simulink model "variable_window_size_alg_1"  (R2019b)
settings: Solver=ode45  StartTime=0.0  StopTime=3  MaxStep=1e-4  RelTol=1e-4  AbsTol=1e-6
values from neighbouring files (symbols this model uses):
  den = [1]    [dab1.m]
  dx = 0    [dab1.m]
  num = [1]    [dab1.m]
libraries: elements x1, simulink x1, simulink_extras x1
settings Model: ExtModeTrigMode=oneshot  ExtModeArmWhenConnect=off  Creator=PC  LastModifiedBy=bae_rashid
settings SolverCC: AutoScaleAbsTol=off
settings DataIOCC: SaveFormat=Array  ReturnWorkspaceOutputs=off
settings OptimizationCC: BlockReduction=off  BooleanDataType=off  LifeSpan=inf
settings DebuggingCC: SaveWithParameterizedLinksMsg=none  UnderspecifiedInitializationDetection=Classic  MergeDetectMultiDrivingBlocksExec=none  SignalResolutionControl=TryResolveAllWithWarning  MultiTaskDSMMsg=warning  MultiTaskCondExecSysMsg=none  SFUnexpectedBacktrackingDiag=warning  SFNoUnconditionalDefaultTransitionDiag=warning  SFExecutionAtInitializationDiag=none  ArithmeticOperatorsInVariantConditions=warning
settings HardwareCC: ProdBitPerPointer=32  ProdBitPerSizeT=32  ProdBitPerPtrDiffT=32  ProdLargestAtomicFloat=None  ProdIntDivRoundTo=Undefined  ProdEndianess=Unspecified  ProdWordSize=32  ProdHWDeviceType=32-bit Generic  TargetUnknown=on
settings ModelReferenceCC: PropagateSignalLabelsOutOfModel=off
settings SFSimCC: SimUseLocalCustomCode=off  CustomCodeUndefinedFunction=UseInterfaceOnly
settings RTWCC: TemplateMakefile=grt_vc.tmf  RTWUseLocalCustomCode=off
settings CodeAppCC: StateflowObjectComments=on
settings GRTTargetCC: TargetLangStandard=C89/C90 (ANSI)  GeneratePreprocessorConditionals=Disable all  CombineOutputUpdateFcns=off  GRTInterface=on
settings ConfigComp: CovMetricSettings=dw  CovHtmlReporting=on  CovSaveCumulativeToWorkspaceVar=on  CovSaveSingleToWorkspaceVar=on  CovExternalEMLEnable=off

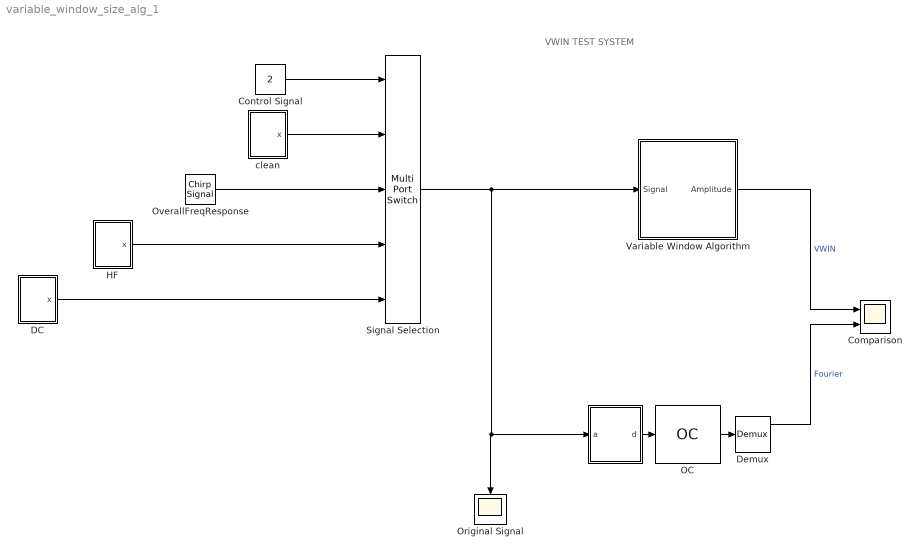
== system variable_window_size_alg_1 ==
  note: VWIN TEST SYSTEM
  "  " : Subsystem  mask(Data Adquisition Board){filter=on, approx=Butterworth, order=3, numerator=[], denominator=[], freq=180, resdis=on, vertres=8, xmax=100, winsize=60, G=1.0, fs=60*60}
      mask prompts: filter "Disable Analog Filter"; approx "Filter approximation"; numerator "Free expression filter: numerator(descending order of s)"; denominator "Free expression filter: denominator:"; freq "Cut-off frequency"; resdis "Disable Vertical Resolution"; vertres "Vertical Resolution: No. of bits"; xmax "Vertical Resolution: signal range"; winsize "Window size"; G "Gain"; fs "Sampling frequency"
      mask help: Takes the instantaneous value of the input signal and convert it to the data window of samples.
      mask init:
      | dab1
      mask TypeOptions approx: Bessel | Tschebyscheff | Butterworth | free expression
      mask TypeOptions order: 2 | 3 | 4
      mask TypeOptions vertres: 8 | 12 | 16
      mask Display: disp('DAB')
  Comparison : Scope  NumInputPorts=2
  Control Signal : Constant  Value=2
  DC : Subsystem  mask(Signal Generator){A1=10, f1=60, A2=0, f2=2*60, A3=0, f3=5*60, tstart=1.5/60, phase1=pi/4*1, bias=5}
      mask prompts: A1 "Amplitude 1"; f1 "Frequency 1 [Hz]"; A2 "Amplitude 2"; f2 "Frequency 2 [Hz]"; A3 "Amplitude 3"; f3 "Frequency 3 [Hz]"; tstart "Start time [sec]"; phase1 "Phase 1"
  Demux : Demux  Outputs=2
  HF : Subsystem  mask(Signal Generator){A1=10, f1=60, A2=3, f2=2*60, A3=2, f3=3*60, tstart=1.5/60, phase1=pi/4*1, bias=0}
      mask prompts: A1 "Amplitude 1"; f1 "Frequency 1 [Hz]"; A2 "Amplitude 2"; f2 "Frequency 2 [Hz]"; A3 "Amplitude 3"; f3 "Frequency 3 [Hz]"; tstart "Start time [sec]"; phase1 "Phase 1"
  OC : elements/OC  tfilt=Fourier  rfilt=[ ]  ifilt=[ ]  tlen=half  N1=60
  Original Signal : Scope
  OverallFreqResponse : simulink/Sources/Chirp Signal  f1=0  T=3  f2=180
  Signal Selection : MultiPortSwitch  Inputs=4
  Variable Window Algorithm : Subsystem  mask{sr=60*60, ws_start=60, ws_end=60, t_switch=0.2}
      mask prompts: sr "Sampling Rate [Hz]"; ws_start "Initial Window Size [# of Samples]"; ws_end "Final Window Size [# of Samples]"; t_switch "Time to extend window [sec]"
  clean : Subsystem  mask(Signal Generator){A1=10, f1=60, A2=0, f2=2*60, A3=0, f3=5*60, tstart=1.5/60, phase1=pi/4*1, bias=0}
      mask prompts: A1 "Amplitude 1"; f1 "Frequency 1 [Hz]"; A2 "Amplitude 2"; f2 "Frequency 2 [Hz]"; A3 "Amplitude 3"; f3 "Frequency 3 [Hz]"; tstart "Start time [sec]"; phase1 "Phase 1"
  wires:
  Control Signal/1 -> Signal Selection/1
  clean/1(x) -> Signal Selection/2
  OverallFreqResponse/1 -> Signal Selection/3
  HF/1(x) -> Signal Selection/4
  DC/1(x) -> Signal Selection/5
  "  "/1(d) -> OC/1
  OC/1 -> Demux/1
  Demux/1 -> Comparison/2  "Fourier"
  Signal Selection/1 -> Original Signal/1, "  "/1(a), Variable Window Algorithm/1(Signal)
  Variable Window Algorithm/1(Amplitude) -> Comparison/1  "VWIN"

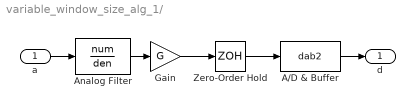
== system variable_window_size_alg_1/   ==
  a : Inport
  A/D & Buffer : S-Function  FunctionName=dab2  Parameters=winsize,fs,dx,resdis  SFunctionDeploymentMode=off  EnableBusSupport=off
  Analog Filter : TransferFcn  Numerator=num  Denominator=den
  Gain : Gain  Gain=G  SaturateOnIntegerOverflow=on  OutDataTypeStr=Inherit: Same as input  ParamDataTypeStr=Inherit: Same as input
  Zero-Order Hold : ZeroOrderHold  SampleTime=1/fs
  d : Outport  InitialOutput=[zeros(winsize,1)]
  wires:
  Analog Filter/1 -> Gain/1
  Gain/1 -> Zero-Order Hold/1
  Zero-Order Hold/1 -> A/D & Buffer/1
  a/1 -> Analog Filter/1
  A/D & Buffer/1 -> d/1

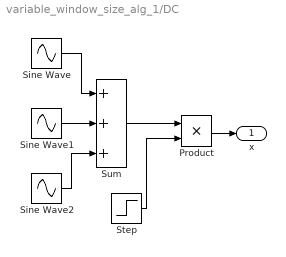
== system variable_window_size_alg_1/DC ==
  Product : Product  SaturateOnIntegerOverflow=on  RndMeth=Zero  InputSameDT=on  OutDataTypeStr=Inherit: Same as first input
  Sine Wave : Sin  Amplitude=A1  Bias=bias  Frequency=f1*2*pi  Phase=phase1  SampleTime=0
  Sine Wave1 : Sin  Amplitude=A2  Bias=bias  Frequency=f2*2*pi  Phase=phase1  SampleTime=0
  Sine Wave2 : Sin  Amplitude=A3  Bias=bias  Frequency=f3*2*pi  Phase=phase1  SampleTime=0
  Step : Step  Time=tstart
  Sum : Sum  Inputs=+++  SaturateOnIntegerOverflow=on  InputSameDT=on  OutDataTypeStr=Inherit: Same as first input
  x : Outport  InitialOutput=0
  wires:
  Sine Wave/1 -> Sum/1
  Sine Wave1/1 -> Sum/2
  Sine Wave2/1 -> Sum/3
  Sum/1 -> Product/1
  Step/1 -> Product/2
  Product/1 -> x/1

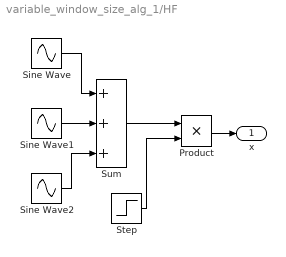
== system variable_window_size_alg_1/HF ==
  Product : Product  SaturateOnIntegerOverflow=on  RndMeth=Zero  InputSameDT=on  OutDataTypeStr=Inherit: Same as first input
  Sine Wave : Sin  Amplitude=A1  Bias=bias  Frequency=f1*2*pi  Phase=phase1  SampleTime=0
  Sine Wave1 : Sin  Amplitude=A2  Bias=bias  Frequency=f2*2*pi  Phase=phase1  SampleTime=0
  Sine Wave2 : Sin  Amplitude=A3  Bias=bias  Frequency=f3*2*pi  Phase=phase1  SampleTime=0
  Step : Step  Time=tstart
  Sum : Sum  Inputs=+++  SaturateOnIntegerOverflow=on  InputSameDT=on  OutDataTypeStr=Inherit: Same as first input
  x : Outport  InitialOutput=0
  wires:
  Sine Wave/1 -> Sum/1
  Sine Wave1/1 -> Sum/2
  Sine Wave2/1 -> Sum/3
  Sum/1 -> Product/1
  Step/1 -> Product/2
  Product/1 -> x/1

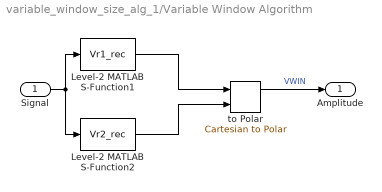
== system variable_window_size_alg_1/Variable Window Algorithm ==
  Signal : Inport
  Level-2 MATLAB S-Function1 : M-S-Function  FunctionName=Vr1_rec  Parameters=sr,ws_start,ws_end,t_switch
  Level-2 MATLAB S-Function2 : M-S-Function  FunctionName=Vr2_rec  Parameters=sr,ws_start,ws_end,t_switch
  to Polar : simulink_extras/Transformations/Cartesian to Polar
      settings: SourceProductName=Simulink
  Amplitude : Outport
  wires:
  Signal/1 -> Level-2 MATLAB S-Function1/1, Level-2 MATLAB S-Function2/1
  Level-2 MATLAB S-Function1/1 -> to Polar/1
  Level-2 MATLAB S-Function2/1 -> to Polar/2
  to Polar/1 -> Amplitude/1  "VWIN"

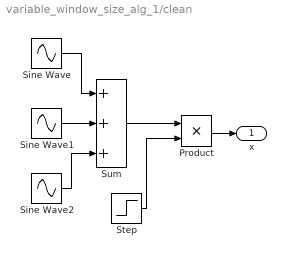
== system variable_window_size_alg_1/clean ==
  Product : Product  SaturateOnIntegerOverflow=on  RndMeth=Zero  InputSameDT=on  OutDataTypeStr=Inherit: Same as first input
  Sine Wave : Sin  Amplitude=A1  Bias=bias  Frequency=f1*2*pi  Phase=phase1  SampleTime=0
  Sine Wave1 : Sin  Amplitude=A2  Bias=bias  Frequency=f2*2*pi  Phase=phase1  SampleTime=0
  Sine Wave2 : Sin  Amplitude=A3  Bias=bias  Frequency=f3*2*pi  Phase=phase1  SampleTime=0
  Step : Step  Time=tstart
  Sum : Sum  Inputs=+++  SaturateOnIntegerOverflow=on  InputSameDT=on  OutDataTypeStr=Inherit: Same as first input
  x : Outport  InitialOutput=0
  wires:
  Sine Wave/1 -> Sum/1
  Sine Wave1/1 -> Sum/2
  Sine Wave2/1 -> Sum/3
  Sum/1 -> Product/1
  Step/1 -> Product/2
  Product/1 -> x/1
